simulink model "Prova_UDP"  (R2019b)
settings: Solver=FixedStepDiscrete  StartTime=0.0  StopTime=inf  FixedStep=0.001  RelTol=1e-3
libraries: xpcutilitieslib x2, xpcrtudplib x2, vrlib x1
settings Model: EnablePacing=on  Creator=carlo  LastModifiedBy=carlo

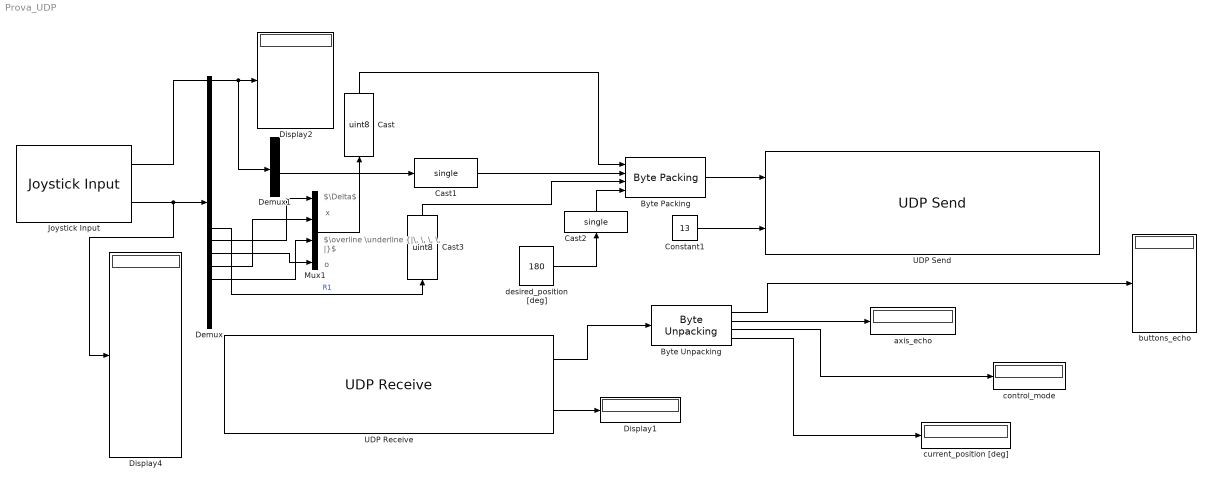
== system Prova_UDP ==
  note: $\overline \underline {|\, \, \, \, |}$
  note: o
  note: $\Delta$
  note: x
  "Byte Packing " : xpcutilitieslib/Byte Packing   MaskPackedDataType=uint8  MaskUnpackedDataTypes={'uint8','single','uint8','single'}  MaskAlignment=1
  "Byte Unpacking " : xpcutilitieslib/Byte Unpacking   MaskUnpackedDataTypes={'uint8','single','uint8','single'}  MaskUnpackedDataSizes={[4],[1],[1],[1]}  MaskAlignment=1
      settings: SourceProductName=Simulink Real-Time  SourceProductBaseCode=XP
  Cast : DataTypeConversion  OutDataTypeStr=uint8
  Cast1 : DataTypeConversion  OutDataTypeStr=single
  Cast2 : DataTypeConversion  OutDataTypeStr=single
  Cast3 : DataTypeConversion  OutDataTypeStr=uint8
  Constant1 : Constant  Value=13
  Demux : Demux  Outputs=19
  Demux1 : Demux
  Display1 : Display
  Display2 : Display
  Display4 : Display
  Joystick Input : vrlib/Joystick Input  joyid=1  adjustports=on  forcefeed=off
      settings: SourceProductName=Simulink
  Mux1 : Mux
  UDP Receive : xpcrtudplib/UDP Receive  ipAddressVal=Use host-target connection  localPort=11111  rcvWidth=13  rcvFmAny=on  fmAddress=0.0.0.0  rcvMulticast=off  multicastAddress={}  maxUDPQueue=8  sampleTime=0.01
      settings: SourceProductName=Simulink Real-Time
  UDP Send : xpcrtudplib/UDP Send  ipAddressVal=Use host-target connection  localPort=25001  toAddress=192.168.0.10  toPort=9999  sampleTime=0.01
      settings: SourceProductName=Simulink Real-Time  SourceProductBaseCode=XP
  axis_echo : Display
  buttons_echo : Display
  control_mode : Display
  current_position [deg] : Display
  desired_position [deg] : Constant  Value=180
  wires:
  "Byte Packing "/1 -> UDP Send/1
  UDP Receive/1 -> "Byte Unpacking "/1
  UDP Receive/2 -> Display1/1
  Constant1/1 -> UDP Send/2
  "Byte Unpacking "/2 -> axis_echo/1
  "Byte Unpacking "/3 -> control_mode/1
  "Byte Unpacking "/1 -> buttons_echo/1
  Joystick Input/1 -> Demux1/1, Display2/1
  Joystick Input/2 -> Display4/1, Demux/1
  Demux/15 -> Mux1/2
  Demux/13 -> Mux1/1
  Mux1/1 -> Cast/1
  Cast/1 -> "Byte Packing "/1
  Demux1/3 -> Cast1/1
  Demux/16 -> Mux1/3
  Cast1/1 -> "Byte Packing "/2
  "Byte Unpacking "/4 -> current_position [deg]/1
  Demux/14 -> Mux1/4
  desired_position [deg]/1 -> Cast2/1
  Cast2/1 -> "Byte Packing "/4
  Demux/12 -> Cast3/1  "R1"
  Cast3/1 -> "Byte Packing "/3
